simulink model "AnaModelFault003"  (R2018b)
settings: Solver=VariableStepAuto  StartTime=0.0  StopTime=1.5  MaxStep=1e-4  RelTol=1e-3
values from neighbouring files (symbols this model uses):
  J = 0.275e-3    (= 0.000275)    [StateSpace.m]    (also in init_AnaModel003.m)
  Ki = 1    [init_AnaModel003.m]
  Kp = 0.05    [init_AnaModel003.m]
  L0 = Ll + 1.5*Lms    (= 0.00130602)    [StateSpace.m]    (also in init_AnaModel003.m)
  L1 = Ll + 1.5*Lms    [AnaModel.m]    (also in StateSpace.m = (sqrt(3)* Llm + 1.5 *Lms); init_AnaModel003.m = (sqrt(3)* Llm + 1.5 *Lms))
  L2 = (sqrt(3)/2)*Lms + Llm    [AnaModel.m]    (also in StateSpace.m = 0.0010375; init_AnaModel003.m = 0.0010375)
  P = 6    [StateSpace.m]    (also in init_AnaModel003.m)
  Phi_f = 0.03    [StateSpace.m]    (also in init_AnaModel003.m)
  rs = 1.98    [StateSpace.m]    (also in init_AnaModel003.m)
  Tm = 1    [StateSpace.m]    (also in init_AnaModel003.m)
libraries: powerlib x48, powerlib_meascontrol x9, simulink x7
(part 2 of 2)

== system AnaModelFault003/Supply and control/PWM Switching Signals for Phase 2/Subsystem2 ==
  In1 : Inport
  Constant : Constant  Value=0.5
  Product : Product
  Sum : Sum  Inputs=|++
  Sum1 : Sum  Inputs=|+-
  Out1 : Outport
  Out2 : Outport  Port=2
  wires:
  Sum1/1 -> Out2/1
  Sum/1 -> Out1/1
  Constant/1 -> Sum1/2, Sum/2, Product/2
  In1/1 -> Product/1
  Product/1 -> Sum1/1, Sum/1

== system AnaModelFault003/Supply and control/PWM Switching Signals for Phase 3 /Subsystem ==
  In1 : Inport
  Constant : Constant  Value=0.5
  Product : Product
  Sum : Sum  Inputs=|++
  Sum1 : Sum  Inputs=|+-
  Out1 : Outport
  Out2 : Outport  Port=2
  wires:
  Sum1/1 -> Out2/1
  Sum/1 -> Out1/1
  Constant/1 -> Sum1/2, Sum/2, Product/2
  In1/1 -> Product/1
  Product/1 -> Sum1/1, Sum/1

== system AnaModelFault003/Supply and control/PWM Switching Signals for Phase 3 /Subsystem1 ==
  In1 : Inport
  Constant : Constant  Value=0.5
  Product : Product
  Sum : Sum  Inputs=|++
  Sum1 : Sum  Inputs=|+-
  Out1 : Outport
  Out2 : Outport  Port=2
  wires:
  Product/1 -> Sum/1, Sum1/1
  In1/1 -> Product/1
  Constant/1 -> Product/2, Sum/2, Sum1/2
  Sum/1 -> Out1/1
  Sum1/1 -> Out2/1

== system AnaModelFault003/Supply and control/PWM Switching Signals for Phase 3 /Subsystem2 ==
  In1 : Inport
  Constant : Constant  Value=0.5
  Product : Product
  Sum : Sum  Inputs=|++
  Sum1 : Sum  Inputs=|+-
  Out1 : Outport
  Out2 : Outport  Port=2
  wires:
  Sum1/1 -> Out2/1
  Sum/1 -> Out1/1
  Constant/1 -> Sum1/2, Sum/2, Product/2
  In1/1 -> Product/1
  Product/1 -> Sum1/1, Sum/1

== system AnaModelFault003/Supply and control/PWM Switching Signals for Phase1 1/Subsystem ==
  In1 : Inport
  Constant : Constant  Value=0.5
  Product : Product
  Sum : Sum  Inputs=|++
  Sum1 : Sum  Inputs=|+-
  Out1 : Outport
  Out2 : Outport  Port=2
  wires:
  Sum1/1 -> Out2/1
  Sum/1 -> Out1/1
  Constant/1 -> Sum1/2, Sum/2, Product/2
  In1/1 -> Product/1
  Product/1 -> Sum1/1, Sum/1

== system AnaModelFault003/Supply and control/PWM Switching Signals for Phase1 1/Subsystem1 ==
  In1 : Inport
  Constant : Constant  Value=0.5
  Product : Product
  Sum : Sum  Inputs=|++
  Sum1 : Sum  Inputs=|+-
  Out1 : Outport
  Out2 : Outport  Port=2
  wires:
  Product/1 -> Sum/1, Sum1/1
  In1/1 -> Product/1
  Constant/1 -> Product/2, Sum/2, Sum1/2
  Sum/1 -> Out1/1
  Sum1/1 -> Out2/1

== system AnaModelFault003/Supply and control/PWM Switching Signals for Phase1 1/Subsystem2 ==
  In1 : Inport
  Constant : Constant  Value=0.5
  Product : Product
  Sum : Sum  Inputs=|++
  Sum1 : Sum  Inputs=|+-
  Out1 : Outport
  Out2 : Outport  Port=2
  wires:
  Sum1/1 -> Out2/1
  Sum/1 -> Out1/1
  Constant/1 -> Sum1/2, Sum/2, Product/2
  In1/1 -> Product/1
  Product/1 -> Sum1/1, Sum/1

== matlab function AnaModelFault003/abc to dq voltage transform/MATLAB Function1 ==
  data: Va1 input; Val_1 output; Vb1 input; Vc1 input; Vbt_1 output
function [Val_1,Vbt_1] = fcn(Va1, Vb1, Vc1)

T1 = 2/3*[ 1   -0.5       -0.5;
           0   -sqrt(3)/2  sqrt(3)/2;
           0.5  0.5        0.5];
       
Vab = T1*[Va1;Vb1;Vc1];
Val_1 = Vab(1,1);
Vbt_1 = Vab(2,1);

== matlab function AnaModelFault003/MATLAB Function ==
  data: Idq1 input size=[2 1]; idq1_dot output size=[2 1]; Idq2 input size=[2 1]; Idq3 input size=[2 1]; Vdq input size=[6 1]; rs input; L0 input; L1 input; L2 input; Phi_f input; omg input; idq2_dot output size=[2 1]; idq3_dot output size=[2 1]
function [idq1_dot, idq2_dot, idq3_dot ] = fcn(Idq1, Idq2, Idq3, Vdq, rs, L0, L1,L2, Phi_f, omg)

Mat1 = [L0 0 L1 0 L2 0; 
        0 L0 0 L1 0 L2;
        L1 0 L0 0 L1 0;
        0 L1 0 L0 0 L1;
        L2 0 L1 0 L0 0;
        0 L2 0 L1 0 L0];
Mat2 = [-rs -omg*L0 0 -omg*L1 0 -omg*L2;
        omg*L0 -rs omg*L1 0 omg*L2 0;
        0 -omg*L1 -rs -omg*L0 0 -omg*L1;
        omg*L1 0 omg*L0 -rs omg*L1 0;
        0 -omg*L2 0 -omg*L1 -rs -omg*L0;
        omg*L2 0 omg*L1 0 omg*L0 -rs];
Mat3 = [ 1;0;1;0;1;0];
Temp1 = Mat2*[Idq1; Idq2; Idq3];
Temp2 = Phi_f*omg*Mat3;
Temp3 = Vdq + Temp1-Temp2;
Idq_dot = inv(Mat1)*Temp3;
idq1_dot = Idq_dot(1:2,:);
idq2_dot = Idq_dot(3:4,:);
idq3_dot = Idq_dot(5:6,:);

== matlab function AnaModelFault003/abc to dq voltage transform/MATLAB Function2 ==
  data: Va2 input; Val_2 output; Vb2 input; Vc2 input; Vbt_2 output
function [Val_2,Vbt_2] = fcn(Va2, Vb2, Vc2)

T2 = 2/3*[sqrt(3)/2 -sqrt(3)/2 0;
          -0.5 -0.5 1;
          0.5 0.5 0.5];
       
Vab = T2*[Va2;Vb2;Vc2];
Val_2 = Vab(1,1);
Vbt_2 = Vab(2,1);

== matlab function AnaModelFault003/abc to dq voltage transform/MATLAB Function3 ==
  data: Va3 input; Val_3 output; Vb3 input; Vc3 input; Vbt_3 output
function [Val_3,Vbt_3] = fcn(Va3, Vb3, Vc3)

T3 = 2/3*[0.5 -1 0.5;
         -sqrt(3)/2 0 sqrt(3)/2;
         0.5 0.5 0.5];  
       
Vab = T3*[Va3;Vb3;Vc3];
Val_3 = Vab(1,1);
Vbt_3 = Vab(2,1);

== matlab function AnaModelFault003/abc to dq voltage transform/MATLAB Function4 ==
  data: Val input; Vd output; Vbt input; Tht input; Vq output
function [Vd,Vq] = fcn(Val, Vbt, Tht)

T = [cos(Tht) -sin(Tht); sin(Tht) cos(Tht)];
       
Vdq = T*[Val;Vbt];
Vd = Vdq(1,1);
Vq = Vdq(2,1);

== matlab function AnaModelFault003/abc to dq voltage transform/MATLAB Function5 ==
  data: Val input; Vd output; Vbt input; Tht input; Vq output
function [Vd,Vq] = fcn(Val, Vbt, Tht)

T = [cos(Tht) -sin(Tht); sin(Tht) cos(Tht)];
       
Vdq = T*[Val;Vbt];
Vd = Vdq(1,1);
Vq = Vdq(2,1);

== matlab function AnaModelFault003/abc to dq voltage transform/MATLAB Function6 ==
  data: Val input; Vd output; Vbt input; Tht input; Vq output
function [Vd,Vq] = fcn(Val, Vbt, Tht)

T = [cos(Tht) -sin(Tht); sin(Tht) cos(Tht)];
       
Vdq = T*[Val;Vbt];
Vd = Vdq(1,1);
Vq = Vdq(2,1);

== matlab function AnaModelFault003/MATLAB Function1 ==
  data: Idq1 input; Te output; Idq2 input; Idq3 input; Phi_f input; P input
function Te = fcn(Idq1, Idq2, Idq3, Phi_f, P)

Te = -1.5*0.5*P*(Phi_f*(Idq1(1,1)+Idq2(1,1)+Idq3(1,1)));

== matlab function AnaModelFault003/Supply and control/DQ to abc conversion /MATLAB Function2 ==
  data: Val_1 input; Va output; Vbt_1 input; Vb output; Vc output
function [Va, Vb, Vc ] = fcn(Val_1,Vbt_1)

T1 = 2/3*[ 1   -0.5       -0.5;
           0   -sqrt(3)/2  sqrt(3)/2;
           0.5  0.5        0.5];
       
Vabc = inv(T1)*[Val_1;Vbt_1;0];
Va = Vabc(1,1);
Vb = Vabc(2,1);
Vc = Vabc(3,1);

== matlab function AnaModelFault003/Supply and control/DQ to abc conversion /MATLAB Function5 ==
  data: Vd input; Va output; Vq input; Tht input; Vb output
function [Va, Vb] = fcn(Vd,Vq, Tht)

T = [cos(Tht) -sin(Tht); sin(Tht) cos(Tht)];
       
Vab = inv(T)*[Vq;Vd];
Va = Vab(1,1);
Vb = Vab(2,1);

== matlab function AnaModelFault003/Supply and control/DQ to abc conversion /MATLAB Function1 ==
  data: Val_1 input; Va output; Vbt_1 input; Vb output; Vc output
function [Va, Vb, Vc ] = fcn(Val_1,Vbt_1)

T2 = 2/3*[sqrt(3)/2 -sqrt(3)/2 0;
          -0.5 -0.5 1;
          0.5 0.5 0.5];
       
Vabc = inv(T2)*[Val_1;Vbt_1;0];
Va = Vabc(1,1);
Vb = Vabc(2,1);
Vc = Vabc(3,1);

== matlab function AnaModelFault003/Supply and control/DQ to abc conversion /MATLAB Function3 ==
  data: Val_1 input; Va output; Vbt_1 input; Vb output; Vc output
function [Va, Vb, Vc ] = fcn(Val_1,Vbt_1)


T3 = 2/3*[0.5 -1 0.5;
         -sqrt(3)/2 0 sqrt(3)/2;
         0.5 0.5 0.5];  
       
Vabc = inv(T3)*[Val_1;Vbt_1;0];
Va = Vabc(1,1);
Vb = Vabc(2,1);
Vc = Vabc(3,1);

== matlab function AnaModelFault003/Supply and control/DQ to abc conversion /MATLAB Function4 ==
  data: Vd input; Va output; Vq input; Tht input; Vb output
function [Va, Vb] = fcn(Vd,Vq, Tht)

T = [cos(Tht) -sin(Tht); sin(Tht) cos(Tht)];
       
       
Vab = inv(T)*[Vq;Vd];
Va = Vab(1,1);
Vb = Vab(2,1);

== matlab function AnaModelFault003/Supply and control/DQ to abc conversion /MATLAB Function6 ==
  data: Vd input; Va output; Vq input; Tht input; Vb output
function [Va, Vb] = fcn(Vd,Vq, Tht)

T = [cos(Tht) -sin(Tht); sin(Tht) cos(Tht)];
       
       
Vab = inv(T)*[Vq;Vd];
Va = Vab(1,1);
Vb = Vab(2,1);

== matlab function AnaModelFault003/Phase 1 ==
  data: Ial_1 input; Ia output; Ibt_1 input; Ib output; Ic output
function [Ia, Ib, Ic ] = fcn(Ial_1,Ibt_1)

T1 = 2/3*[ 1   -0.5       -0.5;
           0   -sqrt(3)/2  sqrt(3)/2;
           0.5  0.5        0.5];
       
Vabc = inv(T1)*[Ial_1;Ibt_1;0];
Ia = Vabc(1,1);
Ib = Vabc(2,1);
Ic = Vabc(3,1);

== matlab function AnaModelFault003/MATLAB Function5 ==
  data: Id input; Ia output; Iq input; Tht input; Ib output
function [Ia, Ib] = fcn(Id,Iq, Tht)

T = [cos(Tht) -sin(Tht); sin(Tht) cos(Tht)];
       
Vab = inv(T)*[Iq;Id];
Ia = Vab(1,1);
Ib = Vab(2,1);

== matlab function AnaModelFault003/MATLAB Function3 ==
  data: Id input; Ia output; Iq input; Tht input; Ib output
function [Ia, Ib] = fcn(Id,Iq, Tht)

T = [cos(Tht) -sin(Tht); sin(Tht) cos(Tht)];
       
Vab = inv(T)*[Iq;Id];
Ia = Vab(1,1);
Ib = Vab(2,1);

== matlab function AnaModelFault003/Phase 2 ==
  data: Ial_1 input; Ia output; Ibt_1 input; Ib output; Ic output
function [Ia, Ib, Ic ] = fcn(Ial_1,Ibt_1)


   T2 = 2/3*[sqrt(3)/2 -sqrt(3)/2 0;
          -0.5 -0.5 1;
          0.5 0.5 0.5];    
Vabc = inv(T2)*[Ial_1;Ibt_1;0];
Ia = Vabc(1,1);
Ib = Vabc(2,1);
Ic = Vabc(3,1);

== matlab function AnaModelFault003/Phase 3 ==
  data: Ial_1 input; Ia output; Ibt_1 input; Ib output; Ic output
function [Ia, Ib, Ic ] = fcn(Ial_1,Ibt_1)


   T3 = 2/3*[0.5 -1 0.5;
         -sqrt(3)/2 0 sqrt(3)/2;
         0.5 0.5 0.5];  
Vabc = inv(T3)*[Ial_1;Ibt_1;0];
Ia = Vabc(1,1);
Ib = Vabc(2,1);
Ic = Vabc(3,1);

== matlab function AnaModelFault003/MATLAB Function7 ==
  data: Id input; Ia output; Iq input; Tht input; Ib output
function [Ia, Ib] = fcn(Id,Iq, Tht)

T = [cos(Tht) -sin(Tht); sin(Tht) cos(Tht)];
       
Vab = inv(T)*[Iq;Id];
Ia = Vab(1,1);
Ib = Vab(2,1);
